simulink model "vfControlDraft"  (R2024a)
settings: Solver=VariableStepAuto  StartTime=0.0  StopTime=1  RelTol=1e-3
libraries: spsIGBTDiodeLib x6, spsSeriesRLCBranchLib x6, simulink x3, spsAsynchronousMachinepuUnitsLib x1, spsDCVoltageSourceLib x1, spsGroundLib x1, spsSawtoothGeneratorLib x1, spsTHDLib x1, spsThreePhaseParallelRLCBranchLib x1, spsThreePhaseVIMeasurementLib x1, spspowerguiLib x1
settings Model: Creator=farza  LastModifiedBy=farza
settings DataIOCC: ReturnWorkspaceOutputs=off

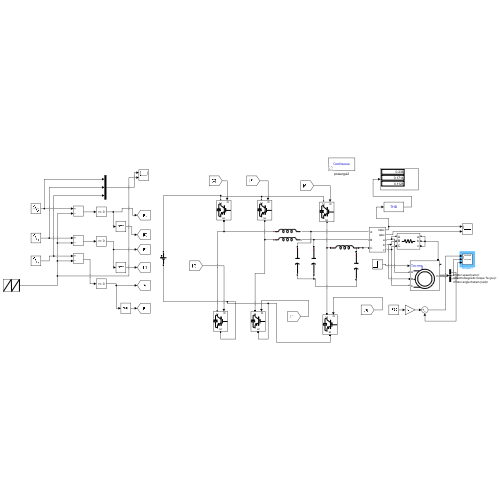
[thumbnail: Simulink's stored preview of the top-level diagram]
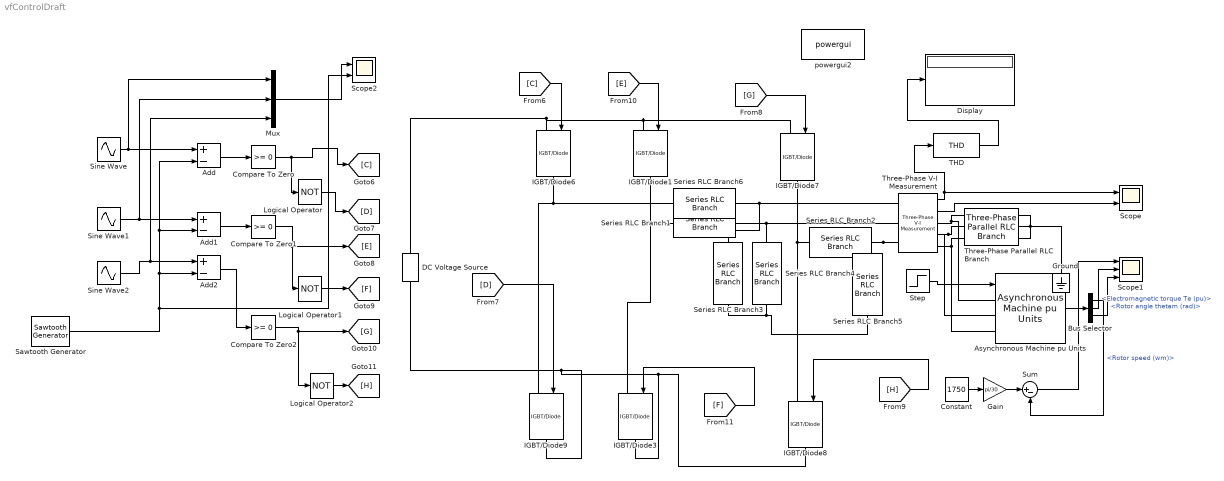
== system vfControlDraft ==
  Add : Sum  Inputs=+-
  Add1 : Sum  Inputs=+-
  Add2 : Sum  Inputs=+-
  Asynchronous Machine pu Units : spsAsynchronousMachinepuUnitsLib/Asynchronous Machine pu Units  RotorType=Squirrel-cage  PresetModel="01:  5 HP   460 V 60Hz 1750 RPM"  MechanicalLoad=Torque Tm  ShowDetailedParameters=on  ReferenceFrame=Rotor  Units=pu  MeasurementBus=off  NominalParameters=[3730 460 60]  VoltageRatio=1  Stator=[0.01965 0.0397]  Rotor=[0.01909 0.0397]  Cage1=[0.01909 0.0397]  Cage2=[0.01909 0.0397]  Lm=1.354  Mechanical=[0.09526 0.05479 2]  PolePairs=2  InitialConditions="[ 1,0   0,0,0   0,0,0 ]"  SimulateSaturation=off  Saturation="[0.212,0.4201,0.8125,1.0979,1.4799,2.2457,3.2586,4.5763,6.4763 ;   0.5,0.7,0.9,1,1.1,1.2 ,1.3,1.4,1.5]"  LoadFlowParameters=0  TsPowergui=0  TsBlock=-1  IterativeModel=Trapezoidal non iterative  IterativeDiscreteModel=Trapezoidal non iterative  Pmec=0
      settings: LibrarySourceBlock=|
      | sps_lib/Electrical Machines/Asynchronous Machine
      | pu Units
  Bus Selector : BusSelector  OutputSignals=Mechanical.Rotor speed (wm),Mechanical.Electromagnetic torque Te (pu),Mechanical.Rotor angle thetam (rad)
  Compare To Zero : simulink/Logic and Bit Operations/Compare To Zero  relop=>=  OutDataTypeStr=boolean
  Compare To Zero1 : simulink/Logic and Bit Operations/Compare To Zero  relop=>=  OutDataTypeStr=boolean
  Compare To Zero2 : simulink/Logic and Bit Operations/Compare To Zero  relop=>=  OutDataTypeStr=boolean
  Constant : Constant  Value=1750
  DC Voltage Source : spsDCVoltageSourceLib/DC Voltage Source  Amplitude=600  Measurements=None
  Display : Display
  Gain : Gain  Gain=pi/30
  Ground : spsGroundLib/Ground  LConnTagsString=a
  IGBT/Diode{1,3,6..9} (6 alike) : spsIGBTDiodeLib/IGBT//Diode  Ron=1e-3  Rs=1e5  Cs=inf  Measurements=off
  Logical Operator : Logic  Operator=NOT  AllPortsSameDT=off  OutDataTypeStr=boolean
  Logical Operator1 : Logic  Operator=NOT  AllPortsSameDT=off  OutDataTypeStr=boolean
  Logical Operator2 : Logic  Operator=NOT  AllPortsSameDT=off  OutDataTypeStr=boolean
  Mux : Mux  Inputs=3
  Sawtooth Generator : spsSawtoothGeneratorLib/Sawtooth Generator  Freq=5000  Phase=0  Ts=0
  Scope : Scope  NumInputPorts=2
  Scope1 : Scope  NumInputPorts=3
  Scope2 : Scope  NumInputPorts=2
  Series RLC Branch1 : spsSeriesRLCBranchLib/Series RLC Branch  LConnTagsString=__new0  RConnTagsString=__new0  BranchType=L  Resistance=1  Inductance=2e-3  SetiL0=off  InitialCurrent=0  Capacitance=1e-6  Setx0=off  InitialVoltage=0  Measurements=None
  Series RLC Branch2 : spsSeriesRLCBranchLib/Series RLC Branch  LConnTagsString=__new0  RConnTagsString=__new0  BranchType=L  Resistance=1  Inductance=2e-3  SetiL0=off  InitialCurrent=0  Capacitance=1e-6  Setx0=off  InitialVoltage=0  Measurements=None
  Series RLC Branch3 : spsSeriesRLCBranchLib/Series RLC Branch  LConnTagsString=__new0  RConnTagsString=__new0  BranchType=C  Resistance=1  Inductance=1e-3  SetiL0=off  InitialCurrent=0  Capacitance=20e-6  Setx0=off  InitialVoltage=0  Measurements=None
  Series RLC Branch4 : spsSeriesRLCBranchLib/Series RLC Branch  LConnTagsString=__new0  RConnTagsString=__new0  BranchType=C  Resistance=1  Inductance=1e-3  SetiL0=off  InitialCurrent=0  Capacitance=20e-6  Setx0=off  InitialVoltage=0  Measurements=None
  Series RLC Branch5 : spsSeriesRLCBranchLib/Series RLC Branch  LConnTagsString=__new0  RConnTagsString=__new0  BranchType=C  Resistance=1  Inductance=1e-3  SetiL0=off  InitialCurrent=0  Capacitance=20e-6  Setx0=off  InitialVoltage=0  Measurements=None
  Series RLC Branch6 : spsSeriesRLCBranchLib/Series RLC Branch  LConnTagsString=__new0  RConnTagsString=__new0  BranchType=L  Resistance=1  Inductance=2e-3  SetiL0=off  InitialCurrent=0  Capacitance=1e-6  Setx0=off  InitialVoltage=0  Measurements=None
  Sine Wave : Sin  Frequency=2*pi*50  SampleTime=0
  Sine Wave1 : Sin  Frequency=2*pi*50  Phase=120  SampleTime=0
  Sine Wave2 : Sin  Frequency=2*pi*50  Phase=-120  SampleTime=0
  Step : Step  Time=5  SampleTime=0
  Sum : Sum  Inputs=|+-
  THD : spsTHDLib/THD  Freq=60  Ts=0
  Three-Phase Parallel RLC Branch : spsThreePhaseParallelRLCBranchLib/Three-Phase Parallel RLC Branch  LConnTagsString=A|B|C  RConnTagsString=A|B|C  BranchType=R  Resistance=60  Inductance=1e-3  Capacitance=1e-6  Measurements=None
  Three-Phase V-I Measurement : spsThreePhaseVIMeasurementLib/Three-Phase V-I Measurement  VoltageMeasurement=phase-to-phase  SetLabelV=off  LabelV=Vabc  Vpu=off  VpuLL=off  CurrentMeasurement=yes  SetLabelI=off  LabelI=Iabc  Ipu=off  Pbase=100e6  Vbase=500e3  OutputType=Complex  PhasorSimulation=off  PSBequivalent=0
  powergui2 : spspowerguiLib/powergui  Priority=1  SimulationMode=Continuous  SampleTime=50e-6  frequency=60  Iterations=50  frequencyindice=0  Pbase=100e6  ErrMax=1e-4  UnitsV=kV  UnitsW=MW  buscounter=0  FunctionMessages=off  echomessages=off  EnableUseOfTLC=off  CurrentSourceSwitches=off  DisableSnubberDevices=off  DisableRonSwitches=off  DisableVfSwitches=off  DisplayEquations=off  AutomaticDiscreteSolvers=off  SolverType=Tustin/Backward Euler (TBE)  Interpol=off  ExternalGateDelay=off  methode=off  Ts=100  x0status=blocks  SPID=on  SwTol=0  HookPort=off  NonlinearTolerance=0  nMaxIteration=15  ContinueOnMaxIteration=off  RestoreLinks=warning  ResistiveCurrentMeasurement=off  Frange=[0:2:500]  Ylog=off  Xlog=on  ShowGrid=off  save=off  variable=ZData  structure=0  ZoomFFT=off  StartTime=0.0  cycles=1  DisplayStyle=1  fundamental=60  FreqAxis=off  MaxFrequency=1000  frequencyindicesteady=1  RmsSteady=1  display=off
  wires:
  Add/1 -> Compare To Zero/1
  [D] -> IGBT/Diode9/1
  Sawtooth Generator/1 -> Scope2/2, Add2/2, Add/2, Add1/2
  Compare To Zero/1 -> Logical Operator/1, [C]
  [F] -> IGBT/Diode3/1
  Add2/1 -> Compare To Zero2/1
  Compare To Zero1/1 -> Logical Operator1/1, [E]
  [E] -> IGBT/Diode1/1
  Compare To Zero2/1 -> Logical Operator2/1, [G]
  Mux/1 -> Scope2/1
  THD/1 -> Display/1
  [H] -> IGBT/Diode8/1
  [C] -> IGBT/Diode6/1
  [G] -> IGBT/Diode7/1
  Logical Operator/1 -> [D]
  Sine Wave/1 -> Add/1, Mux/1
  Sine Wave1/1 -> Mux/2, Add1/1
  Logical Operator1/1 -> [F]
  Logical Operator2/1 -> [H]
  Three-Phase V-I Measurement/1 -> THD/1, Scope/1
  Sine Wave2/1 -> Mux/3, Add2/1
  Add1/1 -> Compare To Zero1/1
  Three-Phase V-I Measurement/2 -> Scope/2
  Step/1 -> Asynchronous Machine pu Units/1
  Asynchronous Machine pu Units/1 -> Bus Selector/1
  Bus Selector/2 -> Scope1/2  "<Electromagnetic torque Te (pu)>"
  Bus Selector/3 -> Scope1/3  "<Rotor angle thetam (rad)>"
  Bus Selector/1 -> Sum/2  "<Rotor speed (wm)>"
  Constant/1 -> Gain/1
  Gain/1 -> Sum/1
  Sum/1 -> Scope1/1
  connections:
  IGBT/Diode6/LConn1 -- DC Voltage Source/RConn1 -- IGBT/Diode1/LConn1 -- IGBT/Diode7/LConn1
  Three-Phase Parallel RLC Branch/LConn3 -- Asynchronous Machine pu Units/LConn3 -- Three-Phase V-I Measurement/RConn3
  Three-Phase Parallel RLC Branch/LConn2 -- Asynchronous Machine pu Units/LConn2 -- Three-Phase V-I Measurement/RConn2
  Three-Phase V-I Measurement/LConn1 -- Series RLC Branch6/RConn1 -- Series RLC Branch3/LConn1
  IGBT/Diode3/LConn1 -- IGBT/Diode1/RConn1 -- Series RLC Branch1/LConn1
  Three-Phase V-I Measurement/LConn2 -- Series RLC Branch1/RConn1 -- Series RLC Branch4/LConn1
  Series RLC Branch4/RConn1 -- Series RLC Branch3/RConn1 -- Series RLC Branch5/RConn1
  IGBT/Diode8/LConn1 -- IGBT/Diode7/RConn1 -- Series RLC Branch2/LConn1
  IGBT/Diode8/RConn1 -- DC Voltage Source/LConn1 -- IGBT/Diode9/RConn1 -- IGBT/Diode3/RConn1
  Three-Phase Parallel RLC Branch/LConn1 -- Asynchronous Machine pu Units/LConn1 -- Three-Phase V-I Measurement/RConn1
  IGBT/Diode6/RConn1 -- IGBT/Diode9/LConn1 -- Series RLC Branch6/LConn1
  Three-Phase Parallel RLC Branch/RConn3 -- Three-Phase Parallel RLC Branch/RConn1 -- Ground/LConn1 -- Three-Phase Parallel RLC Branch/RConn2
  Three-Phase V-I Measurement/LConn3 -- Series RLC Branch2/RConn1 -- Series RLC Branch5/LConn1
